simulink model "dc_voltage_source"  (R2023a)
settings: configuration reference "config" (kept outside this file)
model workspace (MAT data in the model file):
  dc_voltage_base = Simulink.Parameter
  dc_voltage_base.Value = 48
  dc_voltage_base.Description = '母线电压 基准电压 V'
  dc_voltage_base.DataType = 'single'
  dc_voltage_base.Complexity = 'real'
  dc_voltage_base.Dimensions = [1 1]
  dc_voltage_noise = Simulink.Parameter
  dc_voltage_noise.Value = 0.3
  dc_voltage_noise.Description = '母线电压 电压噪声峰值 V'
  dc_voltage_noise.DataType = 'single'
  dc_voltage_noise.Complexity = 'real'
  dc_voltage_noise.Dimensions = [1 1]
settings Model: DataDictionary=model_config.sldd  ParameterArgumentNames=dc_voltage_base,dc_voltage_noise  Creator=huangcheng  LastModifiedBy=Administrator
settings ConfigSetRef: SourceName=config

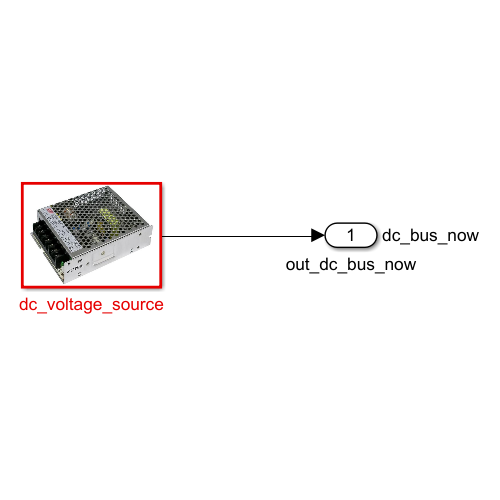
[thumbnail: Simulink's stored preview of the top-level diagram]
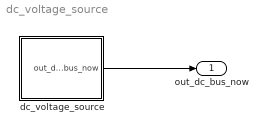
== system dc_voltage_source ==
  dc_voltage_source : Subsystem  TreatAsAtomicUnit=on
      mask Display: image('$imagefile'); % 使用工具条上的 "编辑图像" 进行更改。
  out_dc_bus_now : Outport  SignalName=dc_bus_now  OutDataTypeStr=single
  wires:
  dc_voltage_source/1(out_dc_bus_now) -> out_dc_bus_now/1

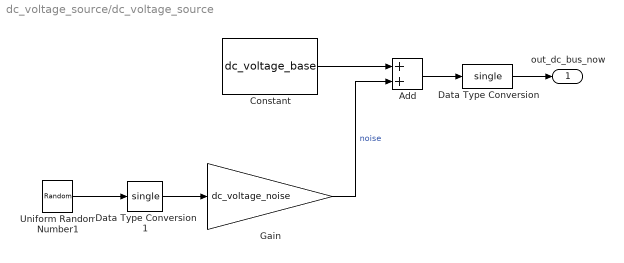
== system dc_voltage_source/dc_voltage_source ==
  Add : Sum
  Constant : Constant  Value=dc_voltage_base  SampleTime=-1
  Data Type Conversion : DataTypeConversion  OutDataTypeStr=single  SaturateOnIntegerOverflow=off  RndMeth=Floor
  Data Type Conversion1 : DataTypeConversion  OutDataTypeStr=single  SaturateOnIntegerOverflow=off  RndMeth=Floor
  Gain : Gain  Gain=dc_voltage_noise
  Uniform Random Number1 : UniformRandomNumber
  out_dc_bus_now : Outport  OutDataTypeStr=single
  wires:
  Add/1 -> Data Type Conversion/1
  Constant/1 -> Add/1
  Uniform Random Number1/1 -> Data Type Conversion1/1
  Data Type Conversion/1 -> out_dc_bus_now/1
  Data Type Conversion1/1 -> Gain/1
  Gain/1 -> Add/2  "noise"
